simulink model "FIR_AsymmetricStream_Ex1"  (R2025a)
settings: Solver=VariableStepAuto  StartTime=0.0  StopTime=1  RelTol=1e-3
PostLoadFcn:
  | % All frequency values are in Hz.
  | Fs = 50000;  % Sampling Frequency
  | Fpass = 5000;              % Passband Frequency
  | Fstop = 10000;             % Stopband Frequency
  | Dpass = 0.0046051376314;   % Passband Ripple
  | Dstop = 0.00025118864315;  % Stopband Attenuation
  | dens  = 16;                % Density Factor
  | % Calculate the order from the parameters using FIRPMORD.
  | [N, Fo, Ao, W] = firpmord([Fpass, Fstop]/(Fs/2), [1 0], [Dpass, Dstop]);
  | % Calculate the coefficients using the FIRPM function.
  | coeffs = firpm(N, Fo, Ao, W, {dens});
undefined symbols (not defined in the file): designMultirateFIR, None, S, vsva2197, xcvc1902
libraries: aieDSP x1, dspsrcs4 x1, dspmlti4 x1, vmcUtilities x1
settings Model: Creator=sdegala  LastModifiedBy=robg
settings ModelReferenceCC: EnableRefExpFcnMdlSchedulingChecks=on
settings RTWCC: GPUComputeCapability=3.5

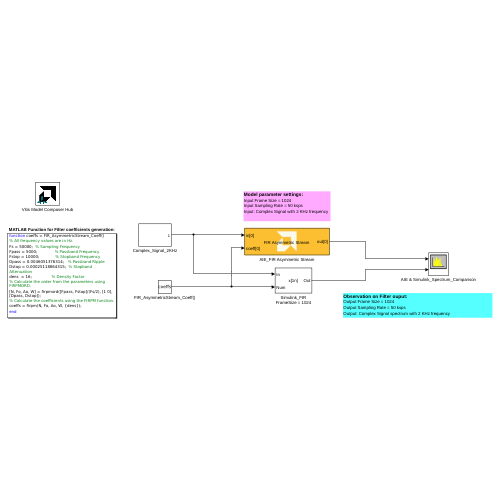
[thumbnail: Simulink's stored preview of the top-level diagram]
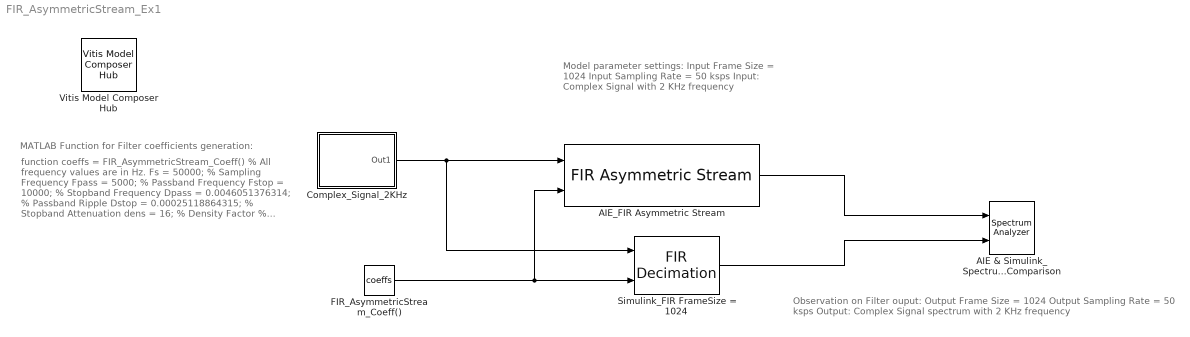
== system FIR_AsymmetricStream_Ex1 ==
  note: function coeffs = FIR_AsymmetricStream_Coeff()
      | % All frequency values are in Hz.
      | Fs = 50000; % Sampling Frequency
      | Fpass = 5000; % Passband Frequency
      | Fstop = 10000; % Stopband Frequency
      | Dpass = 0.0046051376314; % Passband Ripple
      | Dstop = 0.00025118864315; % Stopband Attenuation
      | dens = 16; % Density Factor
      | % Calculate the order from the parameters using FIRPMORD.
      | [N, Fo, Ao, W] = firpmord([Fpass, Fstop]/(Fs/2), [1 0], [Dpass, Dstop]);
      | % Calculate the coefficients using the FIRPM function.
      | coeffs = firpm(N, Fo, Ao, W, {dens});
      | end
  note: Observation on Filter ouput:
      | Output Frame Size = 1024
      | Output Sampling Rate = 50 ksps
      | Output: Complex Signal spectrum with 2 KHz frequency
  note: Model parameter settings:
      | Input Frame Size = 1024
      | Input Sampling Rate = 50 ksps
      | Input: Complex Signal with 2 KHz frequency
  note: MATLAB Function for Filter coefficients generation:
  AIE & Simulink_Spectrum_Comparison : SpectrumAnalyzer  NumInputPorts=2  WindowPosition=[]  AveragingMethod=Exponential  ShowLegend=on  ChannelNames="[\"\"]"  AllowFFTLengthLessThanSamplesPerUpdate=on  DefaultConfigurationName=spbscopes.SpectrumAnalyzerBlockCfg
  AIE_FIR Asymmetric Stream : aieDSP/FIR Asymmetric Stream  data_type=cfloat  coef_type=float  use_coeff_reload=on  dual_ip=off  num_outputs=off  coeff=32  fir_length=32  input_window_size=1024  shift_val=0  rnd_mode=Round to positive infinity  sat_mode=0-None  ssr=1  casc_length=4  AIE_VARIANT=1  TP_API=1  blockJsonConstraints=[]  blockJsonConstraintsInternal=[]  spec=vmc_stream_fir_sr_asym.json  SerializedMaskParamNames=[]  SerializedMaskParamValues=[]  SerializedMaskParamVisibilities=[]  block_type=FIR Asymmetric Stream  SerializedMaskParamDataypes=typename|typename|uint|uint|uint|coef_type|uint|uint|uint|uint|uint|uint|uint|uint|uint  SerializedMaskParamEnumStrArr=0|0|0|0|0|0|0|0|0|Floor,Ceiling,Round to positive infinity,Round to negative infinity,Round symmetrical to infinity,Round symmetrical to zero,Round convergent to even,Round convergent to odd|0-None,1-Asymmetric,3-Symmetric|0|0|0|0  SerializedMaskParamEnumValArr=0|0|0|0|0|0|0|0|0|0,1,2,3,4,5,6,7|0,1,3|0|0|0|0  SerializedMaskParamVectorArr=0|0|0|0|0|1|0|0|0|0|0|0|0|0|0  SerializedMaskParamKeys=TT_DATA|TT_COEFF|TP_USE_COEFF_RELOAD|TP_DUAL_IP|TP_NUM_OUTPUTS|coeff|TP_FIR_LEN|TP_INPUT_WINDOW_VSIZE|TP_SHIFT|TP_RND|TP_SAT|TP_SSR|TP_CASC_LEN|AIE_VARIANT|TP_API
  Complex_Signal_2KHz : Subsystem
  FIR_AsymmetricStream_Coeff() : Constant  Value=coeffs  OutDataTypeStr=single
  Simulink_FIR FrameSize = 1024 : dspmlti4/FIR Decimation  FilterSource=Input port  h=designMultirateFIR(1,2)  D=1  filtStruct=Direct form  FilterObject=FDECIM  InputProcessing=Columns as channels (frame based)  framing=Enforce single-rate processing  AllowArbitraryInputLength=off  inputOffset=0  outputBufInitCond=0  roundingMode=Floor  overflowMode=off  firstCoeffDataTypeStr=Inherit: Same word length as input  firstCoeffMin=[]  firstCoeffMax=[]  firstCoeffLastDataTypeStr=Inherit: Same word length as input  outputDataTypeStr=Inherit: Same as accumulator  outputMin=[]  outputMax=[]  outputLastDataTypeStr=Inherit: Same as accumulator
  Vitis Model Composer Hub : vmcUtilities/Vitis Model Composer Hub  Tag=genX  CodeGeneration=off  StartColumn=1  NumberOfColumns=1  TargetDirectory=./code  exportDesign=off  analyzeDesign=off  validateDesignOnHw=off  ExportType=AI Engines  IpVendor=xilinx.com  IpLibrary=hls  IpVersion=1.0  IpHWLanguage=Verilog  AieCompilerOptions={}  AieSimulatorOptions={}  CreateTestbench=off  TestbenchStackSize=10  RunRtlSim=off  RunCSim=off  RunAieSim=off  enableSimulationTimeout=on  enableGraphIterations=on  AieSimTimeout=50000  AieGraphIterations=-1  RunAieSimProfiling=off  LaunchVitisAnalyzer=off  PlotOutput=off  RunX86Sim=off  X86SimTimeout=10  GenHwImage=off  GenLibadfXo=off  GenHwValidationCode=off  PlatformType=Not Specified  HwSystemType=Baremetal  HwValidationTarget=hw  ProjDevice=xcvc1902-vsva2197-1LP-e-S  ProjDevicePart=xcvc1902-vsva2197-1LP-e-S  AIEType=AIE  SamplePeriod=-1  ClockFrequency=200  DataPathParallelism=1  xilinxfamily=versalaicore  part=xcvc1902  speed=-1LP-e-S  package=vsva2197  directory=./netlist  testbench=off  incr_netlist=off  synthesis_tool=Vivado  clock_wrapper=Clock Enables  dbl_ovrd=According to Block Masks  dcm_input_clock_period=10  sysclk_period=10  simulink_period=1  eval_field=0  LogFileName=''  NThreads=4
  wires:
  Simulink_FIR FrameSize = 1024/1 -> AIE & Simulink_Spectrum_Comparison/2
  FIR_AsymmetricStream_Coeff()/1 -> AIE_FIR Asymmetric Stream/2, Simulink_FIR FrameSize = 1024/2
  Complex_Signal_2KHz/1(Out1) -> AIE_FIR Asymmetric Stream/1, Simulink_FIR FrameSize = 1024/1
  AIE_FIR Asymmetric Stream/1 -> AIE & Simulink_Spectrum_Comparison/1

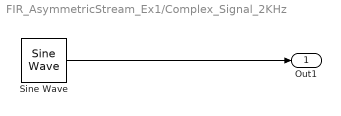
== system FIR_AsymmetricStream_Ex1/Complex_Signal_2KHz ==
  Sine Wave : dspsrcs4/Sine Wave  Amplitude=1  Frequency=2e3  Phase=0  SampleMode=Discrete  OutComplex=Complex  CompMethod=Table lookup  TableSize=Speed  SampleTime=1/50e3  SamplesPerFrame=1024  ResetState=Restart at time zero  OutputFrames=off  dataType=single  wordLen=16  udDataType=sfix(16)  fracBitsMode=User-defined  numFracBits=14  OutDataTypeStr=single  LastOutDataTypeStr=single
  Out1 : Outport
  wires:
  Sine Wave/1 -> Out1/1
